simulink model "dPTPUDPNode4_tm"  (R2018b)
settings: Solver=FixedStepDiscrete  StartTime=0.0  StopTime=inf  FixedStep=0.025  RelTol=1e-3  EnableMultiTasking=on
undefined symbols (not defined in the file): ipaddr, PTP
libraries: ptplib x5, xpcutilitieslib x2, xpcrtudplib x2
settings Model: SimulationMode=external  Creator=The MathWorks, Inc.  LastModifiedBy=MAE-NCSUCORE
settings SolverCC: ConcurrentTasks=on  AutoInsertRateTranBlk=on  DecoupledContinuousIntegration=on  MinimalZcImpactIntegration=on
settings DataIOCC: SaveFormat=StructureWithTime
settings OptimizationCC: BlockReduction=off  OptimizeBlockIOStorage=off  BufferReuse=off  GlobalBufferReuse=off  ExpressionFolding=off  LocalBlockOutputs=off  OptimizeDataStoreBuffers=off  BusAssignmentInplaceUpdate=off
settings DebuggingCC: LibraryContextMissingDiagnostic=none
settings HardwareCC: ProdBitPerPointer=32  ProdBitPerSizeT=32  ProdBitPerPtrDiffT=32  ProdLargestAtomicFloat=None  ProdWordSize=32  ProdLongLongMode=on  ProdHWDeviceType=Generic->32-bit x86 compatible
settings SFSimCC: SimUseLocalCustomCode=off
settings RTWCC: SystemTargetFile=slrt.tlc  TemplateMakefile=slrt_default_tmf  Description=Simulink Real-Time  RTWVerbose=off  RTWUseLocalCustomCode=off  CodeExecutionProfiling=on  RTWCompilerOptimization=on
settings SimulinkRealTimeCC: SupportVariableSizeSignals=on  PreserveStateflowLocalDataDimensions=off  RL32LogTETModifier=off  RL32LogBufSizeModifier=1000000  RL32ObjectName=tg4  xPCisDefaultEnv=off  xPCTargetPCEnvName=Machine5  xPCConcurrentTasks=on

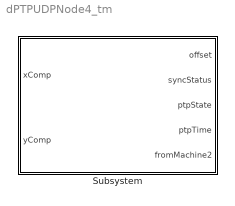
== system dPTPUDPNode4_tm ==
  Subsystem : Subsystem  TreatAsAtomicUnit=on  mask{sample_time=0.025, offset_threshold=250e-6, sync_interval=0.05, min_pdelay_req_interval=0.08, announce_receipt_timeout=10}
      mask prompts: sample_time "Sample time (-1 for inherited)"; offset_threshold "Offset threshold (second)"; sync_interval "Sync interval (second):"; min_pdelay_req_interval "Min delay or pdelay request interval (second):"; announce_receipt_timeout "Announce receipt timeout (in announce intervals):"
      mask TypeOptions sample_time: IEEE 1588 Read Offset/sample_time | IEEE 1588 Read State/sample_time | IEEE 1588 Read Time/sample_time | IEEE 1588 Real-Time UDP/sample_time | IEEE 1588 Sync Status/sample_time | UDP Receive/sampleTime | UDP Send/sampleTime
      mask TypeOptions offset_threshold: IEEE 1588 Sync Status/offset_threshold
      mask TypeOptions sync_interval: IEEE 1588 Real-Time UDP/sync_interval
      mask TypeOptions min_pdelay_req_interval: IEEE 1588 Real-Time UDP/min_pdelay_req_interval
      mask TypeOptions announce_receipt_timeout: IEEE 1588 Real-Time UDP/announce_receipt_timeout

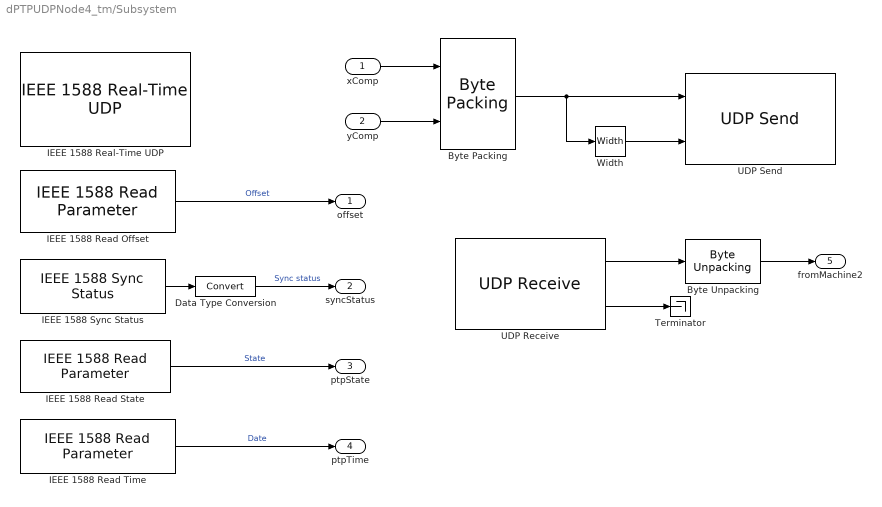
== system dPTPUDPNode4_tm/Subsystem ==
  xComp : Inport
  yComp : Inport  Port=2
  Byte Packing : xpcutilitieslib/Byte Packing   MaskPackedDataType=uint8  MaskUnpackedDataTypes={'double','double'}  MaskAlignment=1
  Byte Unpacking : xpcutilitieslib/Byte Unpacking   MaskUnpackedDataTypes={['uint8']}  MaskUnpackedDataSizes={[3]}  MaskAlignment=1
      settings: SourceProductName=Simulink Real-Time  SourceProductBaseCode=XP
  Data Type Conversion : DataTypeConversion
  IEEE 1588 Read Offset : ptplib/IEEE 1588 Read Parameter  Priority=1  ID=1  param=Offset from Master  sample_time=sample_time  enable_read_precision=off
      settings: SourceProductName=Simulink Real-Time  SourceProductBaseCode=XP
  IEEE 1588 Read State : ptplib/IEEE 1588 Read Parameter  Priority=1  ID=1  param=Protocol state  sample_time=sample_time  enable_read_precision=off
      settings: SourceProductName=Simulink Real-Time  SourceProductBaseCode=XP
  IEEE 1588 Read Time : ptplib/IEEE 1588 Read Parameter  Priority=1  ID=1  param=PTP time (time-of-day)  sample_time=sample_time  enable_read_precision=off
      settings: SourceProductName=Simulink Real-Time  SourceProductBaseCode=XP
  IEEE 1588 Real-Time UDP : ptplib/IEEE 1588 Real-Time UDP  Priority=0  ID=1  PciBus=4  PciSlot=0  PciFunction=0  time_inc=4000000  sample_time=sample_time  IpSource=Specify  IpAddress=30.30.30.3  SubnetMask=255.255.255.0  Gateway=0.0.0.0  Receive1=30.30.30.30  dest_ip_select=Standard PTP multicast (224.0.1.129, 224.0.0.107)  custom_dest_ip_addr=30.30.30.30  MulticastList=[ipaddr('224.0.1.129'), ipaddr('224.0.0.107')]  Multicast={macaddr('01:00:5E:00:01:81'), macaddr('01:00:5E:00:00:6B')}  time_source=Ethernet board  timescale=PTP (1970-01-01)  epoch=[1970 01 01 00]  delay_measure=Request-response  slave_only=off  enable_advanced_config=on  domain_num=0  utc_offset=35  priority1=128  clock_class=248  clock_accuracy=hex2dec('FE')  priority2=128  announce_interval=2  sync_interval=sync_interval  min_pdelay_req_interval=min_pdelay_req_interval  announce_receipt_timeout=announce_receipt_timeout
      settings: SourceProductName=Simulink Real-Time  SourceProductBaseCode=XP
  IEEE 1588 Sync Status : ptplib/IEEE 1588 Sync Status  Priority=1  ID=1  offset_threshold=offset_threshold  sample_time=sample_time
      settings: SourceProductName=Simulink Real-Time  SourceProductBaseCode=XP
  Terminator : Terminator
  UDP Receive : xpcrtudplib/UDP Receive  ipAddressVal=30.30.30.3  localPort=8000  rcvWidth=8  rcvFmAny=off  fmAddress=30.30.30.30  rcvMulticast=off  multicastAddress={}  maxUDPQueue=8  sampleTime=sample_time
      settings: SourceProductName=Simulink Real-Time
  UDP Send : xpcrtudplib/UDP Send  ipAddressVal=30.30.30.3  localPort=-1  toAddress=30.30.30.30  toPort=toPort  sampleTime=sample_time
      settings: SourceProductName=Simulink Real-Time  SourceProductBaseCode=XP
  Width : Width
  offset : Outport
  syncStatus : Outport  Port=2
  ptpState : Outport  Port=3
  ptpTime : Outport  Port=4
  fromMachine2 : Outport  Port=5
  wires:
  Byte Packing/1 -> UDP Send/1, Width/1
  UDP Receive/1 -> Byte Unpacking/1
  Byte Unpacking/1 -> fromMachine2/1
  IEEE 1588 Sync Status/1 -> Data Type Conversion/1
  IEEE 1588 Read Time/1 -> ptpTime/1  "Date"
  IEEE 1588 Read State/1 -> ptpState/1  "State"
  Width/1 -> UDP Send/2
  Data Type Conversion/1 -> syncStatus/1  "Sync status"
  UDP Receive/2 -> Terminator/1
  IEEE 1588 Read Offset/1 -> offset/1  "Offset"
  xComp/1 -> Byte Packing/1
  yComp/1 -> Byte Packing/2
